simulink model "Aufgabe_10_2_4_Umsetzer_und_greifer"  (R2023a)
settings: Solver=ode3  StartTime=0.0  StopTime=10.0  FixedStep=0.01  RelTol=1e-3  EnableMultiTasking=on
libraries: simulink x4
settings Model: Creator=SimTP16  LastModifiedBy=ASUS
settings SolverCC: AlgebraicLoopSolver=TrustRegion
settings DataIOCC: LimitDataPoints=on  SaveFormat=Array  ReturnWorkspaceOutputs=off
settings OptimizationCC: LifeSpan=inf
settings DebuggingCC: UnderspecifiedInitializationDetection=Classic  MergeDetectMultiDrivingBlocksExec=none  SolverPrmCheckMsg=warning  UnconnectedInputMsg=warning  UnconnectedOutputMsg=warning  UnconnectedLineMsg=warning  StateNameClashWarn=warning  SFUnexpectedBacktrackingDiag=warning  SFNoUnconditionalDefaultTransitionDiag=warning  ArithmeticOperatorsInVariantConditions=warning
settings HardwareCC: ProdBitPerPointer=32  ProdBitPerSizeT=32  ProdBitPerPtrDiffT=32  ProdLargestAtomicFloat=None  ProdIntDivRoundTo=Undefined  ProdEndianess=Unspecified  ProdWordSize=32  ProdHWDeviceType=32-bit Generic
settings ModelReferenceCC: EnableRefExpFcnMdlSchedulingChecks=on  PropagateSignalLabelsOutOfModel=off
settings SFSimCC: SimUseLocalCustomCode=off  CustomCodeUndefinedFunction=UseInterfaceOnly
settings RTWCC: RTWUseLocalCustomCode=off
settings CodeAppCC: StateflowObjectComments=on
settings GRTTargetCC: TargetLangStandard=C89/C90 (ANSI)
settings ConfigComp: CovMetricSettings=dw  CovSaveCumulativeToWorkspaceVar=on  CovSaveSingleToWorkspaceVar=on  CovExternalEMLEnable=off

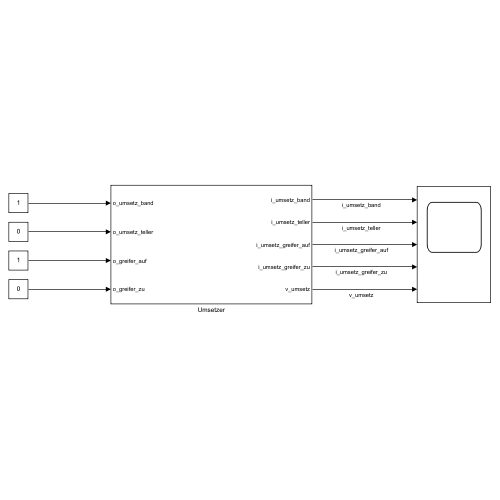
[thumbnail: Simulink's stored preview of the top-level diagram]
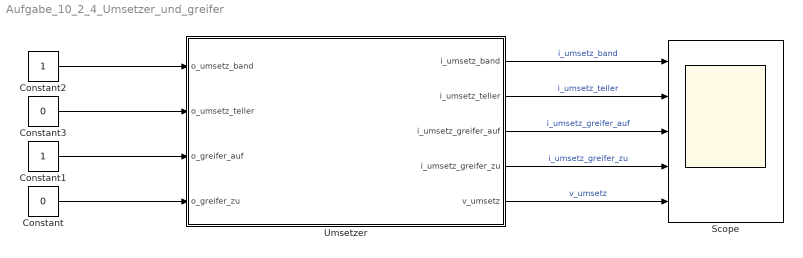
== system Aufgabe_10_2_4_Umsetzer_und_greifer ==
  Constant : Constant  Value=0
  Constant1 : Constant
  Constant2 : Constant
  Constant3 : Constant  Value=0
  Scope : Scope  NumInputPorts=5
  Umsetzer : Subsystem
  wires:
  Constant2/1 -> Umsetzer/1(o_umsetz_band)
  Constant3/1 -> Umsetzer/2(o_umsetz_teller)
  Constant1/1 -> Umsetzer/3(o_greifer_auf)
  Constant/1 -> Umsetzer/4(o_greifer_zu)
  Umsetzer/1(i_umsetz_band) -> Scope/1  "i_umsetz_band"
  Umsetzer/2(i_umsetz_teller) -> Scope/2  "i_umsetz_teller"
  Umsetzer/3(i_umsetz_greifer_auf) -> Scope/3  "i_umsetz_greifer_auf"
  Umsetzer/4(i_umsetz_greifer_zu) -> Scope/4  "i_umsetz_greifer_zu"
  Umsetzer/5(v_umsetz) -> Scope/5  "v_umsetz"

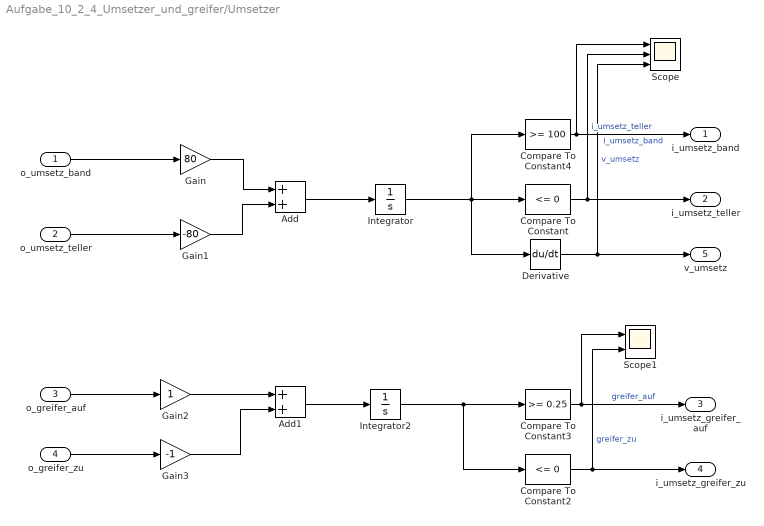
== system Aufgabe_10_2_4_Umsetzer_und_greifer/Umsetzer ==
  o_umsetz_band : Inport
  o_umsetz_teller : Inport  Port=2
  o_greifer_auf : Inport  Port=3
  o_greifer_zu : Inport  Port=4
  Add : Sum
  Add1 : Sum
  Compare To Constant : simulink/Logic and Bit Operations/Compare To Constant  relop=<=  const=0  OutDataTypeStr=boolean
  Compare To Constant2 : simulink/Logic and Bit Operations/Compare To Constant  relop=<=  const=0  OutDataTypeStr=boolean
  Compare To Constant3 : simulink/Logic and Bit Operations/Compare To Constant  relop=>=  const=0.25  OutDataTypeStr=boolean
  Compare To Constant4 : simulink/Logic and Bit Operations/Compare To Constant  relop=>=  const=100  OutDataTypeStr=boolean
  Derivative : Derivative
  Gain : Gain  Gain=80
  Gain1 : Gain  Gain=-80
  Gain2 : Gain
  Gain3 : Gain  Gain=-1
  Integrator : Integrator  LimitOutput=on  UpperSaturationLimit=100  LowerSaturationLimit=0
  Integrator2 : Integrator  LimitOutput=on  UpperSaturationLimit=0.25  LowerSaturationLimit=0
  Scope : Scope  NumInputPorts=3
  Scope1 : Scope  NumInputPorts=2
  i_umsetz_band : Outport
  i_umsetz_teller : Outport  Port=2
  i_umsetz_greifer_auf : Outport  Port=3
  i_umsetz_greifer_zu : Outport  Port=4
  v_umsetz : Outport  Port=5
  wires:
  o_greifer_zu/1 -> Gain3/1
  Gain3/1 -> Add1/2
  Gain2/1 -> Add1/1
  o_umsetz_teller/1 -> Gain1/1
  o_greifer_auf/1 -> Gain2/1
  o_umsetz_band/1 -> Gain/1
  Add1/1 -> Integrator2/1
  Compare To Constant/1 -> Scope/2, i_umsetz_teller/1  "i_umsetz_teller"
  Integrator/1 -> Compare To Constant4/1, Derivative/1, Compare To Constant/1
  Gain/1 -> Add/1
  Gain1/1 -> Add/2
  Add/1 -> Integrator/1
  Derivative/1 -> Scope/3, v_umsetz/1  "v_umsetz"
  Compare To Constant4/1 -> Scope/1, i_umsetz_band/1  "i_umsetz_band"
  Integrator2/1 -> Compare To Constant3/1, Compare To Constant2/1
  Compare To Constant2/1 -> Scope1/2, i_umsetz_greifer_zu/1  "greifer_zu"
  Compare To Constant3/1 -> Scope1/1, i_umsetz_greifer_auf/1  "greifer_auf"
